simulink library "hiToLoElevationControllerExp"  (R2020a)
settings: Solver=VariableStepAuto  StartTime=0.0  StopTime=10.0  RelTol=1e-3
undefined symbols (not defined in the file or in its folder): elSP, env, fltCtrl, initializeBussesFromBlock, vhcl
libraries: ctrlAllocMatrix_cl x1, filteredPIDController_ul x1
settings Model: Creator=jcreed2  LastModifiedBy=Zak

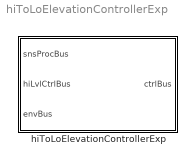
== system hiToLoElevationControllerExp ==
  hiToLoElevationControllerExp : Subsystem  LoadFcn=initializeBussesFromBlock(gcb)  InitFcn=initializeBussesFromBlock(gcb)  StartFcn=initializeBussesFromBlock(gcb)  mask{initPosForInitSStar=vhcl.initPosVecGnd.Value, fluidDensity=env.water.density.Value, pathCtrl=fltCtrl, aeroStruct=vhcl.struct('OCT.aeroSurf'), thrAttach=vhcl.rBridle_LE.Value}
      mask prompts: initPosForInitSStar "Initial Position"; fluidDensity "Fluid Density"; pathCtrl "Controller"; aeroStruct "Aerodynamic Structure"; thrAttach "Tether Attach Point"
      mask DialogControl Container3 Prompt: courseFollow Params
      mask DialogControl Container4 Prompt: setpointToOutput Params

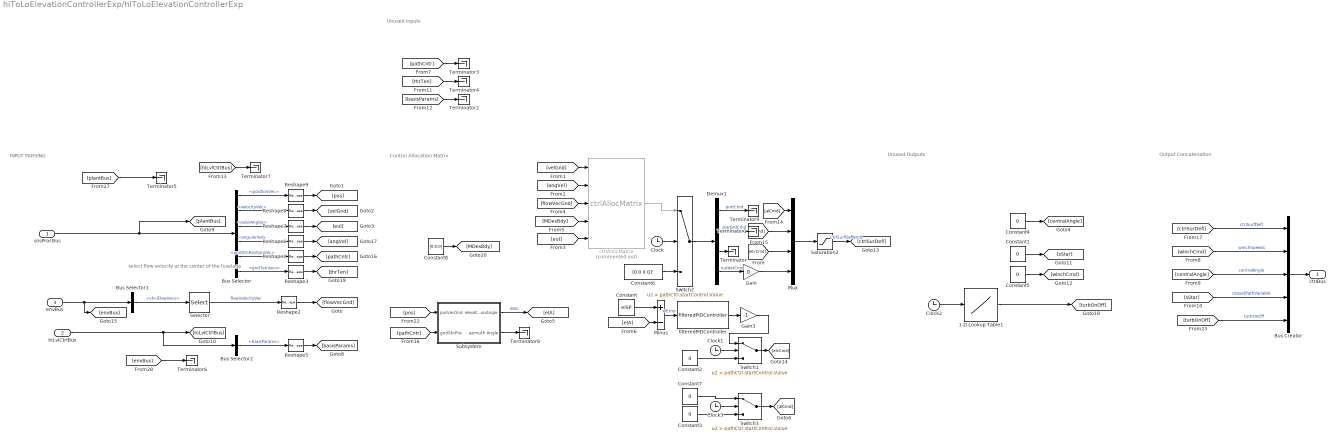
== system hiToLoElevationControllerExp/hiToLoElevationControllerExp ==
  note: Unused Inputs
  note: Control Allocation Matrix
  note: Unused Outputs
  note: INPUT PARSING
  note: select flow velocity at the center of the fuselage
  note: Output Concatenation
  snsProcBus : Inport  OutDataTypeStr=Bus: sensorsProcessingBus
  hiLvlCtrlBus : Inport  Port=2  OutDataTypeStr=Bus: hiLvlCtrlBus
  envBus : Inport  Port=3  OutDataTypeStr=Bus: envBus
  1-D Lookup Table1 : Lookup_n-D  NumberOfTableDimensions=1  BreakpointsForDimension1=[0 1000 2000]  Table=[0 0 0]  InterpMethod=Flat  InternalRulePriority=Speed  RndMeth=Simplest  InputSameDT=on
  Bus Creator : BusCreator  Inputs=5  OutDataTypeStr=Bus: fltCtrlBus
      settings: InheritFromInputs=off
  Bus Selector : BusSelector  OutputSignals=positionVec,velocityVec,eulerAngles,angularVel,gndStnPositionVec,gndTenVecs
  Bus Selector1 : BusSelector  OutputSignals=vhclFlowVecs
  Bus Selector2 : BusSelector  OutputSignals=basisParams
  Clock{,1..3} (4 alike) : Clock
  Constant : Constant  Value=elSP
  Constant{1..5,7} (6 alike) : Constant  Value=0
  Constant6 : Constant  Value=[0 0 0 0]'
  Constant8 : Constant  Value=[0;0;0]
  Demux1 : Demux
  Gain : Gain  Gain=0
  Gain3 : Gain  Gain=-1
  Minus : Sum  Inputs=+-
  Mux : Mux
  Reshape{1..3,5..9} (8 alike) : Reshape  OutputDimensionality=Column vector (2-D)
  Saturation2 : Saturate  UpperLimit=pathCtrl.controlSigMax.upperLimit.Value  LowerLimit=pathCtrl.controlSigMax.lowerLimit.Value
  Selector : Selector  NumberOfDimensions=2  InputPortWidth=3  IndexOptions=Select all,Index vector (dialog)  Indices=[1 3],5  OutputSizes=1,1
  Subsystem : Subsystem  AncestorBlock=pathFollowingController_cl/pathFollowingController/Subsystem
  Switch1 : Switch  Criteria=u2 > Threshold  Threshold=pathCtrl.startControl.Value
  Switch2 : Switch  Criteria=u2 > Threshold  Threshold=pathCtrl.startControl.Value
  Switch3 : Switch  Criteria=u2 > Threshold  Threshold=pathCtrl.startControl.Value
  Terminator{,1..9} (10 alike) : Terminator
  ctrlAllocMatrix : ctrlAllocMatrix_cl/ctrlAllocMatrix  Commented=on  aeroStruct=vhcl.struct('OCT.aeroSurf')  fluidDensity=fluidDensity
  filteredPIDController : filteredPIDController_ul/filteredPIDController  kp=1.5  ki=0  kd=7  Value=.001  externalReset=none
  ctrlBus : Outport  OutDataTypeStr=Bus: fltCtrlBus
  wires:
  Bus Selector/6 -> Reshape3/1  "<gndTenVecs>"
  Reshape3/1 -> [thrTen]
  snsProcBus/1 -> [plantBus], Bus Selector/1
  Bus Selector/2 -> Reshape8/1  "<velocityVec>"
  Bus Selector/1 -> Reshape9/1  "<positionVec>"
  Bus Selector/3 -> Reshape7/1  "<eulerAngles>"
  Reshape9/1 -> [pos]
  Reshape8/1 -> [velGnd]
  Reshape6/1 -> [angVel]
  Reshape7/1 -> [eul]
  Bus Selector/4 -> Reshape6/1  "<angularVel>"
  Bus Selector2/1 -> Reshape5/1  "<basisParams>"
  Bus Selector/5 -> Reshape1/1  "<gndStnPositionVec>"
  Reshape2/1 -> [flowVecGnd]
  Selector/1 -> Reshape2/1  "flowVelocityVec"
  Reshape5/1 -> [basisParams]
  [envBus] -> Terminator6/1
  Bus Selector1/1 -> Selector/1  "<vhclFlowVecs>"
  [plantBus] -> Terminator5/1
  Reshape1/1 -> [pathCntr]
  [centralAngle] -> Bus Creator/3  "centralAngle"
  [ctrlSurDefl] -> Bus Creator/1  "ctrlSurfDefl"
  [sStar] -> Bus Creator/4  "closestPathVariable"
  [turbOnOff] -> Bus Creator/5  "turbOnOff"
  Bus Creator/1 -> ctrlBus/1
  [winchCmd] -> Bus Creator/2  "winchSpeeds"
  1-D Lookup Table1/1 -> [turbOnOff]
  Clock2/1 -> 1-D Lookup Table1/1
  ctrlAllocMatrix/1 -> Switch2/1
  Constant6/1 -> Switch2/3
  Clock/1 -> Switch2/2
  Constant1/1 -> [sStar]
  Constant4/1 -> [centralAngle]
  Constant5/1 -> [winchCmd]
  Saturation2/1 -> [ctrlSurDefl]  "ctrlSurfDeflCmd"
  Switch2/1 -> Demux1/1
  Mux/1 -> Saturation2/1
  Demux1/4 -> Gain/1  "rudderCmd"
  Gain/1 -> Mux/4
  Demux1/1 -> Terminator9/1  "portCmd"
  Demux1/2 -> Terminator1/1  "starBrdCmd"
  Demux1/3 -> Terminator/1
  [velGnd] -> ctrlAllocMatrix/1
  [angVel] -> ctrlAllocMatrix/2
  [eul] -> ctrlAllocMatrix/5
  [flowVecGnd] -> ctrlAllocMatrix/3
  Constant8/1 -> [MDesBdy]
  [MDesBdy] -> ctrlAllocMatrix/4
  [basisParams] -> Terminator2/1
  [pathCntr] -> Terminator3/1
  [thrTen] -> Terminator4/1
  hiLvlCtrlBus/1 -> Bus Selector2/1, [hiLvlCtrlBus]
  envBus/1 -> [envBus], Bus Selector1/1
  [hiLvlCtrlBus] -> Terminator7/1
  Switch1/1 -> [elvCmd]
  Clock1/1 -> Switch1/2
  [elA] -> Minus/2
  Constant2/1 -> Switch1/3
  [pos] -> Subsystem/1(posVecGnd)
  Subsystem/1(elevationAngle) -> [elA]  "elAn"
  Subsystem/2(azimuth Angle) -> Terminator8/1
  Gain3/1 -> Switch1/1
  filteredPIDController/1 -> Gain3/1
  Minus/1 -> filteredPIDController/1  "elError"
  Constant/1 -> Minus/1
  Clock3/1 -> Switch3/2
  Constant3/1 -> Switch3/3
  Constant7/1 -> Switch3/1
  Switch3/1 -> [alCmd]
  [alCmd] -> Mux/1
  [alCmd] -> Mux/2
  [elvCmd] -> Mux/3
  [pathCntr] -> Subsystem/2(gndStnPos)

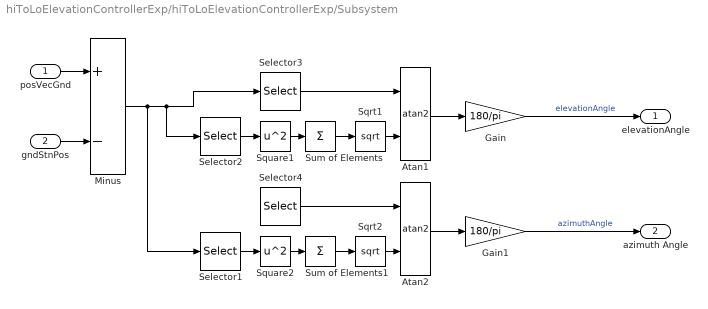
== system hiToLoElevationControllerExp/hiToLoElevationControllerExp/Subsystem ==
  posVecGnd : Inport
  gndStnPos : Inport  Port=2
  Atan1 : Trigonometry  Operator=atan2
  Atan2 : Trigonometry  Operator=atan2
  Gain : Gain  Gain=180/pi
  Gain1 : Gain  Gain=180/pi
  Minus : Sum  Inputs=+-
  Selector1 : Selector  InputPortWidth=3  IndexOptions=Index vector (dialog)  Indices=1  OutputSizes=1
  Selector2 : Selector  InputPortWidth=3  IndexOptions=Index vector (dialog)  Indices=[1 2]  OutputSizes=1
  Selector3 : Selector  InputPortWidth=3  IndexOptions=Index vector (dialog)  Indices=3  OutputSizes=1
  Selector4 : Selector  InputPortWidth=3  IndexOptions=Index vector (dialog)  Indices=2  OutputSizes=1
  Sqrt1 : Sqrt  SaturateOnIntegerOverflow=on
  Sqrt2 : Sqrt  SaturateOnIntegerOverflow=on
  Square1 : Math  Operator=square  SignedPower=on  SaturateOnIntegerOverflow=on
  Square2 : Math  Operator=square  SignedPower=on  SaturateOnIntegerOverflow=on
  Sum of Elements : Sum  Inputs=+
  Sum of Elements1 : Sum  Inputs=+
  elevationAngle : Outport
  azimuth Angle : Outport  Port=2
  wires:
  Gain1/1 -> azimuth Angle/1  "azimuthAngle"
  Selector4/1 -> Atan2/1
  Sqrt2/1 -> Atan2/2
  Selector1/1 -> Square2/1
  Sum of Elements1/1 -> Sqrt2/1
  Square2/1 -> Sum of Elements1/1
  Atan2/1 -> Gain1/1
  Gain/1 -> elevationAngle/1  "elevationAngle"
  Selector2/1 -> Square1/1
  Atan1/1 -> Gain/1
  Sum of Elements/1 -> Sqrt1/1
  Selector3/1 -> Atan1/1
  Square1/1 -> Sum of Elements/1
  Sqrt1/1 -> Atan1/2
  posVecGnd/1 -> Minus/1
  gndStnPos/1 -> Minus/2
  Minus/1 -> Selector1/1, Selector2/1, Selector3/1
